simulink model "Task3_sim"  (R2014a)
settings: Solver=ode45  StartTime=0.0  StopTime=0.3  RelTol=1e-3
settings Model: Creator=bunka  LastModifiedBy=bunka

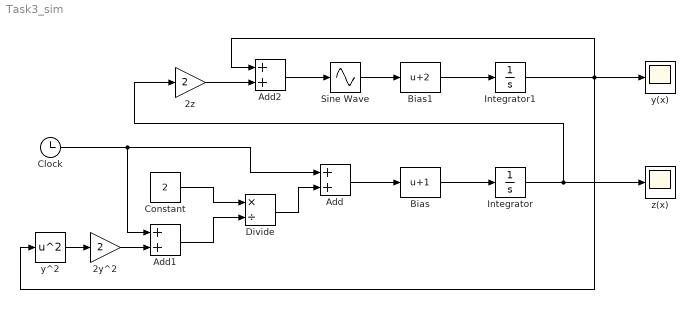
== system Task3_sim ==
  2y^2 : Gain  Gain=2
  2z : Gain  Gain=2
  Add : Sum
  Add1 : Sum
  Add2 : Sum
  Bias : Bias  Bias=1
  Bias1 : Bias  Bias=2
  Clock : Clock
  Constant : Constant  Value=2
  Divide : Product  Inputs=*/
  Integrator : Integrator  InitialCondition=0.05
  Integrator1 : Integrator  InitialCondition=1
  Sine Wave : Sin  TimeSource=Use external signal  Amplitude=-1  Phase=pi/-2  SampleTime=0
  y(x) : Scope
  y^2 : Math  Operator=square  SaturateOnIntegerOverflow=on
  "z(x) " : Scope
  wires:
  Bias/1 -> Integrator/1
  Bias1/1 -> Integrator1/1
  Integrator/1 -> 2z/1, "z(x) "/1
  Integrator1/1 -> y^2/1, Add2/1, y(x)/1
  Add/1 -> Bias/1
  Add1/1 -> Divide/2
  2y^2/1 -> Add1/2
  y^2/1 -> 2y^2/1
  Constant/1 -> Divide/1
  Divide/1 -> Add/2
  Sine Wave/1 -> Bias1/1
  Add2/1 -> Sine Wave/1
  2z/1 -> Add2/2
  Clock/1 -> Add1/1, Add/1
